simulink model "model_obsv_state"  (R2016b)
settings: Solver=ode45  StartTime=0.0  StopTime=12  MaxStep=1e-3  RelTol=1e-3  EnableMultiTasking=on
values from neighbouring files (symbols this model uses):
  A = [ ... (first row only)    [linearize.m]
  B = [ ... (first row only)    [linearize.m]
  C = [1 0 0 0; 0 0 1 0]    [pendulum.m]
  L1 = [831.873247833582,11.2052740269567;173863.136517871,4656.17642490115;8.24339500067234,828.126752165350;3309.70675970819,171351.081489223]    [pendulum.m]
  N_bar = -inv(Cn*((A-B*K1)\B))    [pendulum.m]
undefined symbols (not defined in the file or in its folder): J, Kd, L, m, r
undefined symbols (not defined in the file): M
settings Model: Creator=Patrick  LastModifiedBy=Craig
settings DataIOCC: LimitDataPoints=on  SaveFormat=Array  SignalLoggingSaveFormat=ModelDataLogs
settings OptimizationCC: ExpressionDepthLimit=2147483647  LifeSpan=inf
settings DebuggingCC: UnderspecifiedInitializationDetection=Classic  MergeDetectMultiDrivingBlocksExec=none  SolverPrmCheckMsg=warning  FcnCallInpInsideContextMsg=warning  StateNameClashWarn=warning  SFUnexpectedBacktrackingDiag=warning  SFNoUnconditionalDefaultTransitionDiag=warning  SFExecutionAtInitializationDiag=none
settings HardwareCC: ProdBitPerPointer=32  ProdBitPerSizeT=32  ProdBitPerPtrDiffT=32  ProdLargestAtomicFloat=None  ProdIntDivRoundTo=Undefined  ProdEndianess=Unspecified  ProdWordSize=32  ProdHWDeviceType=32-bit Generic
settings ModelReferenceCC: PropagateSignalLabelsOutOfModel=off
settings GRTTargetCC: TargetLangStandard=C89/C90 (ANSI)  GeneratePreprocessorConditionals=Disable all  CombineOutputUpdateFcns=off  GRTInterface=on
settings ConfigComp: CovMetricSettings=dw  CovHtmlReporting=on  CovSaveCumulativeToWorkspaceVar=on  CovSaveSingleToWorkspaceVar=on  CovExternalEMLEnable=off

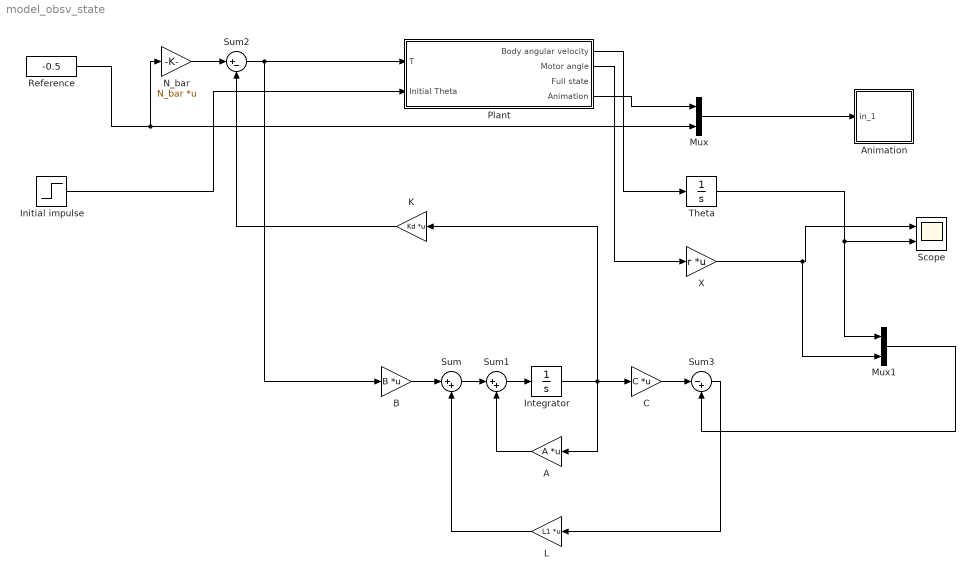
== system model_obsv_state ==
  A : Gain  Gain=A  Multiplication=Matrix(K*u)
  Animation : Subsystem  mask(Pendulum plot){RefBlock=Reference, L=L, r=r, Ts=1e-3}
      mask prompts: RefBlock "DC reference signal block name:"; L "Location of mass"; r "Radius of wheel"; Ts "Simulation time step"
      mask help: Pendulum plot
      mask Help: Pendulum animation function using Handle graphics.
      mask Display: plot([-10 10],[0 0],[-2 -2 2 2],[0 1 1 0],[0 3],[1 5])
  B : Gain  Gain=B  Multiplication=Matrix(K*u)
  C : Gain  Gain=C  Multiplication=Matrix(K*u)
  "Initial impulse " : Step  Time=6  After=0  SampleTime=0
  Integrator : Integrator
  K : Gain  Gain=Kd  Multiplication=Matrix(K*u)
  L : Gain  Gain=L1  Multiplication=Matrix(K*u)
  Mux : Mux  Inputs=2
  Mux1 : Mux  Inputs=2
  N_bar : Gain  Gain=N_bar  Multiplication=Matrix(K*u)
  Plant : Subsystem  mask{m=m, mw=M, J=J, r=r, L=L, g=9.81, theta0=0.1}
      mask prompts: m "Mass of body"; mw "Mass of wheel"; J "Inertia of wheel"; r "Radius of wheel"; L "Height of body COM"; g "Gravity"; theta0 "Initial angle"
  Reference : Constant  Value=-0.5
  Scope : Scope  NumInputPorts=2
  Sum : Sum  Inputs=|++
  Sum1 : Sum  Inputs=|++
  Sum2 : Sum  Inputs=|+-
  Sum3 : Sum  Inputs=|-+
  "Theta " : Integrator
  X : Gain  Gain=r  Multiplication=Matrix(K*u)
  wires:
  Plant/4(Animation) -> Mux/1
  K/1 -> Sum2/2
  A/1 -> Sum1/2
  Sum/1 -> Sum1/1
  B/1 -> Sum/1
  Sum1/1 -> Integrator/1
  Integrator/1 -> A/1, K/1, C/1
  C/1 -> Sum3/1
  Plant/1(Body angular velocity) -> "Theta "/1
  Sum3/1 -> L/1
  L/1 -> Sum/2
  Sum2/1 -> B/1, Plant/1(T)
  Plant/2(Motor angle) -> X/1
  X/1 -> Scope/1, Mux1/2
  "Theta "/1 -> Scope/2, Mux1/1
  Mux1/1 -> Sum3/2
  N_bar/1 -> Sum2/1
  Reference/1 -> Mux/2, N_bar/1
  "Initial impulse "/1 -> Plant/2(Initial Theta)
  Mux/1 -> Animation/1(in_1)

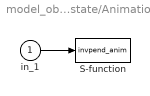
== system model_obsv_state/Animation ==
  in_1 : Inport
  S-function : S-Function  FunctionName=invpend_anim  Parameters=RefBlock,L,r,Ts  SFunctionDeploymentMode=off  EnableBusSupport=off
      settings: DeleteFcn=pendan([],[],[],'DeleteBlock');
  wires:
  in_1/1 -> S-function/1

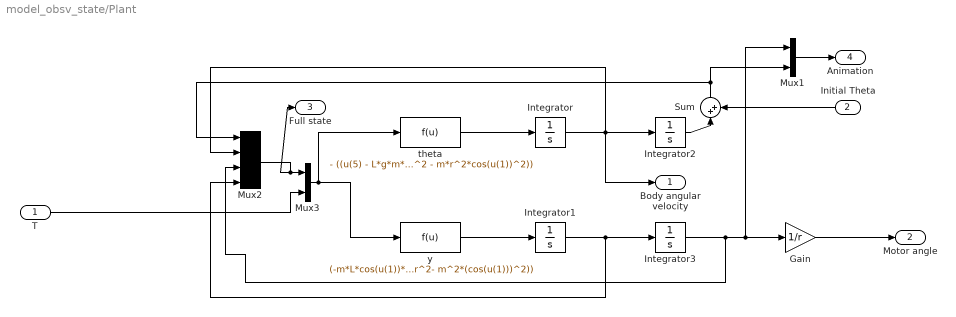
== system model_obsv_state/Plant ==
  T : Inport
  Initial Theta : Inport  Port=2
  Gain : Gain  Gain=1/r
  Integrator{,1..3} (4 alike) : Integrator
  Mux1 : Mux  Inputs=2
  Mux2 : Mux
  Mux3 : Mux  Inputs=2
  Sum : Sum  Inputs=|++
  theta : Fcn  Expr=- ((u(5) - L*g*m*sin(u(1)))*(J + m*r^2 + mw*r^2))/(L^2*m*(J + m*r^2 + mw*r^2 - m*r^2*cos(u(1))^2)) - (r^2*cos(u(1))*(u(5)/r + L*m*u(2)^2*sin(u(1))))/(L*(J + m*r^2 + mw*r^2 - m*r^2*cos(u(1))^2))
  y : Fcn  Expr=(-m*L*cos(u(1))*(m*g*L*sin(u(1)) - u(5)) + m*L^2*(m*L*u(2)^2*sin(u(1))+u(5)/r))/(L^2*(m^2+m*mw+(m*J)/r^2- m^2*(cos(u(1)))^2))
  Body angular velocity : Outport
  Motor angle : Outport  Port=2
  Full state : Outport  Port=3
  Animation : Outport  Port=4
  wires:
  y/1 -> Integrator1/1
  Integrator/1 -> Body angular velocity/1, Integrator2/1, Mux2/2
  Integrator1/1 -> Integrator3/1, Mux2/4
  Integrator3/1 -> Gain/1, Mux1/1, Mux2/3
  T/1 -> Mux3/2
  Gain/1 -> Motor angle/1
  Integrator2/1 -> Sum/1
  Sum/1 -> Mux1/2, Mux2/1
  Initial Theta/1 -> Sum/2
  Mux1/1 -> Animation/1
  Mux2/1 -> Full state/1, Mux3/1
  Mux3/1 -> theta/1, y/1
  theta/1 -> Integrator/1
